simulink model "uavsim"  (R2024b)
settings: Solver=ode23  StartTime=0.0  StopTime=60  RelTol=1e-3  EnableMultiTasking=on
values from neighbouring files (symbols this model uses):
  P = real(.5*P + .5*P')    [ekf_driver.m]    (also in init_uavsim_params.m = []; load_uavsim.m = compute_autopilot_gains(models,P))
undefined symbols (not defined in the file or in its folder): uavsim_control, uavsim_display, uavsim_estimates, uavsim_forces_moments, uavsim_kin_dyn, uavsim_logging, uavsim_sensors, uavsim_trajectory_control, uavsim_truth_feedback, uavsim_wind
libraries: simulink x6
settings Model: Creator=bartojd1  LastModifiedBy=yeboaka1
settings SolverCC: AlgebraicLoopSolver=TrustRegion
settings DataIOCC: LimitDataPoints=on  SaveFormat=Array  SignalLoggingSaveFormat=ModelDataLogs  SaveOutput=off  SignalLogging=off  SaveTime=off  ReturnWorkspaceOutputs=off
settings OptimizationCC: ExpressionDepthLimit=2147483647  LifeSpan=inf
settings DebuggingCC: SolverPrmCheckMsg=warning  FcnCallInpInsideContextMsg=warning  UnconnectedInputMsg=warning  UnconnectedOutputMsg=warning  UnconnectedLineMsg=warning  StateNameClashWarn=warning  SFUnexpectedBacktrackingDiag=warning  SFNoUnconditionalDefaultTransitionDiag=warning  SFExecutionAtInitializationDiag=none  ArithmeticOperatorsInVariantConditions=warning
settings HardwareCC: ProdBitPerPointer=32  ProdBitPerSizeT=32  ProdBitPerPtrDiffT=32  ProdLargestAtomicFloat=None  ProdIntDivRoundTo=Undefined  ProdEndianess=Unspecified  ProdWordSize=32  ProdHWDeviceType=32-bit Generic
settings ModelReferenceCC: PropagateSignalLabelsOutOfModel=off
settings SFSimCC: SimUseLocalCustomCode=off  CustomCodeUndefinedFunction=UseInterfaceOnly
settings RTWCC: RTWUseLocalCustomCode=off  GPUComputeCapability=3.5
settings CodeAppCC: StateflowObjectComments=on
settings GRTTargetCC: TargetLangStandard=C89/C90 (ANSI)  CombineOutputUpdateFcns=off  GRTInterface=on
settings ConfigComp: CovMetricSettings=dw  CovSaveCumulativeToWorkspaceVar=on  CovSaveSingleToWorkspaceVar=on  CovExternalEMLEnable=off  CovSFcnEnable=off

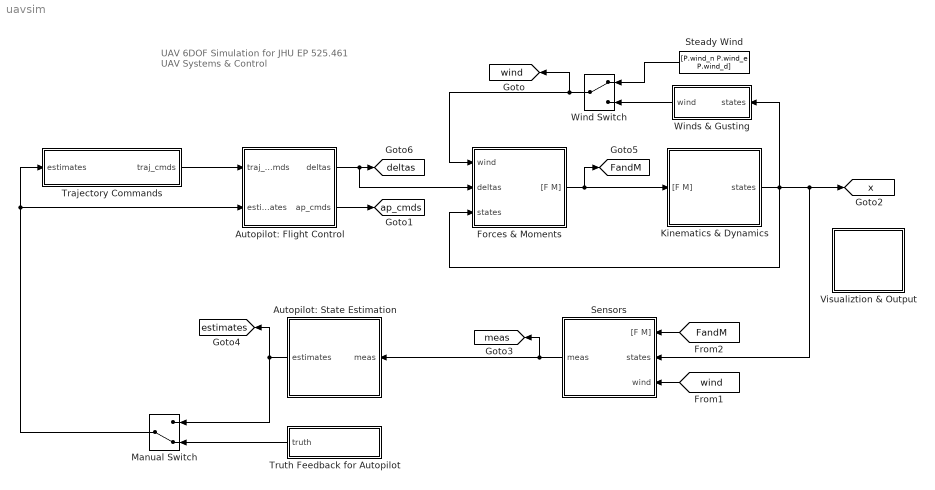
== system uavsim ==
  note: UAV 6DOF Simulation
      | for JHU EP 525.461
      | UAV Systems & Control
  Autopilot: Flight Control : Subsystem
  Autopilot: State Estimation : Subsystem
  Forces & Moments : Subsystem
  Kinematics & Dynamics : Subsystem
  Manual Switch : ManualSwitch  CurrentSetting=0
  Sensors : Subsystem
  Steady Wind : Constant  Value=[P.wind_n P.wind_e P.wind_d]
  Trajectory Commands : Subsystem
  Truth Feedback for Autopilot : Subsystem
  Visualiztion & Output : Subsystem
  Wind Switch : ManualSwitch
  Winds & Gusting : Subsystem
  tag scope: FandM=global, ap_cmds=global, deltas=global, estimates=global, meas=global, wind=global, x=global
  wires:
  Kinematics & Dynamics/1(states) -> Forces & Moments/3(states), Winds & Gusting/1(states), [x], Sensors/2(states)
  Forces & Moments/1("[F M]") -> Kinematics & Dynamics/1("[F M]"), [FandM]
  Sensors/1(meas) -> Autopilot: State Estimation/1(meas), [meas]
  [wind] -> Sensors/3(wind)
  Autopilot: Flight Control/2(ap_cmds) -> [ap_cmds]
  [FandM] -> Sensors/1("[F M]")
  Trajectory Commands/1(" traj_cmds") -> Autopilot: Flight Control/1(traj_cmds)
  Winds & Gusting/1(wind) -> Wind Switch/2
  Wind Switch/1 -> Forces & Moments/1("wind  "), [wind]
  Steady Wind/1 -> Wind Switch/1
  Autopilot: Flight Control/1(deltas) -> [deltas], Forces & Moments/2(deltas)
  Autopilot: State Estimation/1(estimates) -> Manual Switch/1, [estimates]
  Truth Feedback for Autopilot/1(truth) -> Manual Switch/2
  Manual Switch/1 -> Autopilot: Flight Control/2(estimates), Trajectory Commands/1(estimates)

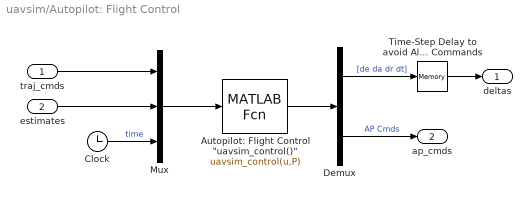
== system uavsim/Autopilot: Flight Control ==
  traj_cmds : Inport
  estimates : Inport  Port=2
  "Autopilot: Flight Control \"uavsim_control()\"" : MATLABFcn  MATLABFcn=uavsim_control(u,P)  OutputDimensions=4+9  SampleTime="P.Ts     % Autopilot at 100Hz"
  Clock : Clock
  Demux : Demux  Outputs=[4;9]
  Mux : Mux  Inputs=3
  Time-Step Delay to avoid Algepraic Loop I.C.: Trim Commands : Memory  InitialCondition=[P.delta_e0 P.delta_a0 P.delta_r0 P.delta_t0]'
  deltas : Outport
  ap_cmds : Outport  Port=2
  wires:
  Clock/1 -> Mux/3  "time"
  "Autopilot: Flight Control \"uavsim_control()\""/1 -> Demux/1
  Mux/1 -> "Autopilot: Flight Control \"uavsim_control()\""/1
  estimates/1 -> Mux/2
  traj_cmds/1 -> Mux/1
  Demux/2 -> ap_cmds/1  "AP Cmds"
  Demux/1 -> Time-Step Delay to avoid Algepraic Loop I.C.: Trim Commands/1  "[de da dr dt]"
  Time-Step Delay to avoid Algepraic Loop I.C.: Trim Commands/1 -> deltas/1

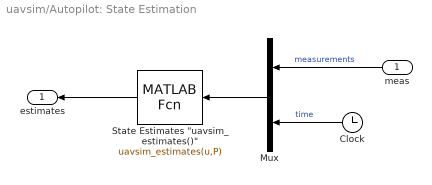
== system uavsim/Autopilot: State Estimation ==
  meas : Inport
  Clock : Clock
  Mux : Mux  Inputs=2
  "State Estimates \"uavsim_estimates()\"" : MATLABFcn  MATLABFcn=uavsim_estimates(u,P)  OutputDimensions=23  SampleTime="P.Ts   % Autopilot at 100 Hz"
  estimates : Outport
  wires:
  meas/1 -> Mux/1  "measurements"
  Mux/1 -> "State Estimates \"uavsim_estimates()\""/1
  Clock/1 -> Mux/2  "time"
  "State Estimates \"uavsim_estimates()\""/1 -> estimates/1

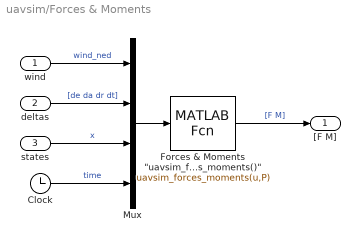
== system uavsim/Forces & Moments ==
  "wind  " : Inport
  deltas : Inport  Port=2
  states : Inport  Port=3
  Clock : Clock
  "Forces & Moments \"uavsim_forces_moments()\"" : MATLABFcn  MATLABFcn=uavsim_forces_moments(u,P)  OutputDimensions=3+3 % (3 forces), (3 moments)
  Mux : Mux
  "[F M]" : Outport
  wires:
  "Forces & Moments \"uavsim_forces_moments()\""/1 -> "[F M]"/1  "[F M]"
  Mux/1 -> "Forces & Moments \"uavsim_forces_moments()\""/1
  Clock/1 -> Mux/4  "time"
  "wind  "/1 -> Mux/1  "wind_ned"
  deltas/1 -> Mux/2  "[de da dr dt]"
  states/1 -> Mux/3  "x"

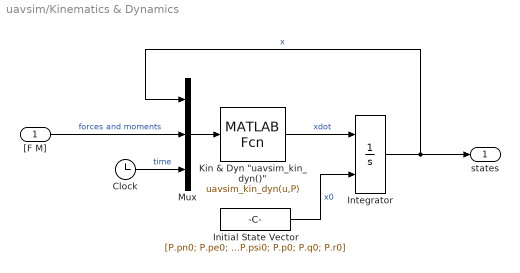
== system uavsim/Kinematics & Dynamics ==
  "[F M]" : Inport
  Clock : Clock
  Initial State Vector : Constant  Value=[P.pn0; P.pe0; P.pd0; P.u0; P.v0; P.w0; P.phi0; P.theta0; P.psi0; P.p0; P.q0; P.r0]
  Integrator : Integrator  InitialConditionSource=external
  "Kin & Dyn \"uavsim_kin_dyn()\"" : MATLABFcn  MATLABFcn=uavsim_kin_dyn(u,P)  OutputDimensions="12    % # of states"
  Mux : Mux  Inputs=3
  states : Outport
  wires:
  Integrator/1 -> Mux/1, states/1  "x"
  Mux/1 -> "Kin & Dyn \"uavsim_kin_dyn()\""/1
  "Kin & Dyn \"uavsim_kin_dyn()\""/1 -> Integrator/1  "xdot"
  "[F M]"/1 -> Mux/2  "forces and moments"
  Initial State Vector/1 -> Integrator/2  "x0"
  Clock/1 -> Mux/3  "time"

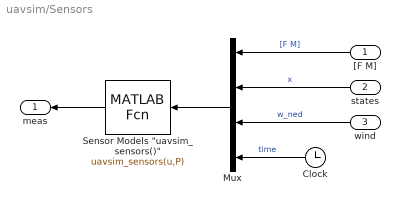
== system uavsim/Sensors ==
  "[F M]" : Inport
  states : Inport  Port=2
  wind : Inport  Port=3
  Clock : Clock
  Mux : Mux
  "Sensor Models \"uavsim_sensors()\"" : MATLABFcn  MATLABFcn=uavsim_sensors(u,P)  OutputDimensions=18  SampleTime=P.Ts
  meas : Outport
  wires:
  Mux/1 -> "Sensor Models \"uavsim_sensors()\""/1
  "Sensor Models \"uavsim_sensors()\""/1 -> meas/1
  Clock/1 -> Mux/4  "time"
  "[F M]"/1 -> Mux/1  "[F M]"
  states/1 -> Mux/2  "x"
  wind/1 -> Mux/3  "w_ned"

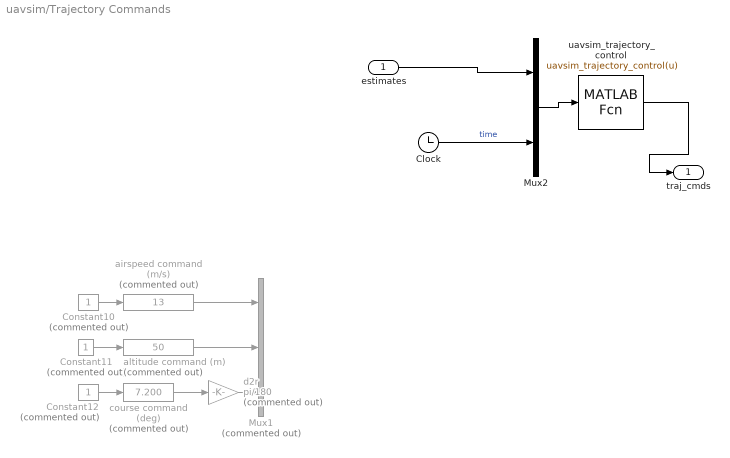
== system uavsim/Trajectory Commands ==
  estimates : Inport
  Clock : Clock
  Constant10 : Constant  Commented=on
  Constant11 : Constant  Commented=on
  Constant12 : Constant  Commented=on
  Mux1 : Mux  Commented=on  Inputs=3
  Mux2 : Mux  Inputs=2
  airspeed command (m/s) : simulink/Math Operations/Slider Gain  Commented=on  gain=13  low=5  high=18
  altitude command (m) : simulink/Math Operations/Slider Gain  Commented=on  gain=50  low=0  high=100
  course command (deg) : simulink/Math Operations/Slider Gain  Commented=on  gain=7.200  low=-360  high=360
  d2r : Gain  Commented=on  Gain=pi/180
  uavsim_trajectory_control : MATLABFcn  MATLABFcn=uavsim_trajectory_control(u)  OutputDimensions=3  SampleTime="P.Ts     % Autopilot at 100Hz"
  " traj_cmds" : Outport
  wires:
  Constant10/1 -> airspeed command (m/s)/1
  Constant11/1 -> altitude command (m)/1
  Constant12/1 -> course command (deg)/1
  course command (deg)/1 -> d2r/1
  altitude command (m)/1 -> Mux1/2
  airspeed command (m/s)/1 -> Mux1/1
  d2r/1 -> Mux1/3
  uavsim_trajectory_control/1 -> " traj_cmds"/1
  estimates/1 -> Mux2/1
  Clock/1 -> Mux2/2  "time"
  Mux2/1 -> uavsim_trajectory_control/1

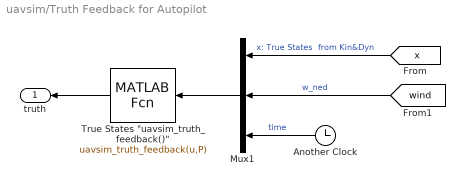
== system uavsim/Truth Feedback for Autopilot ==
  Another Clock : Clock
  Mux1 : Mux  Inputs=3
  "True States \"uavsim_truth_feedback()\"" : MATLABFcn  MATLABFcn=uavsim_truth_feedback(u,P)  OutputDimensions=23  SampleTime="P.Ts   % Autopilot at 100 Hz"
  truth : Outport
  wires:
  Mux1/1 -> "True States \"uavsim_truth_feedback()\""/1
  [x] -> Mux1/1  "x: True States  from Kin&Dyn"
  [wind] -> Mux1/2  "w_ned"
  Another Clock/1 -> Mux1/3  "time"
  "True States \"uavsim_truth_feedback()\""/1 -> truth/1

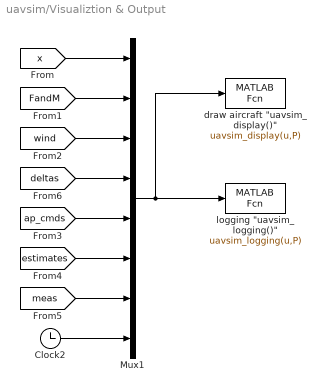
== system uavsim/Visualiztion & Output ==
  Clock2 : Clock
  Mux1 : Mux  Inputs=8
  "draw aircraft \"uavsim_display()\"" : MATLABFcn  MATLABFcn=uavsim_display(u,P)  OutputDimensions=0  SampleTime=P.Tvis
  "logging \"uavsim_logging()\"" : MATLABFcn  MATLABFcn=uavsim_logging(u,P)  OutputDimensions=0  SampleTime=P.Tlog
  wires:
  [FandM] -> Mux1/2
  [wind] -> Mux1/3
  Mux1/1 -> "logging \"uavsim_logging()\""/1, "draw aircraft \"uavsim_display()\""/1
  [x] -> Mux1/1
  [deltas] -> Mux1/4
  [ap_cmds] -> Mux1/5
  [estimates] -> Mux1/6
  [meas] -> Mux1/7
  Clock2/1 -> Mux1/8

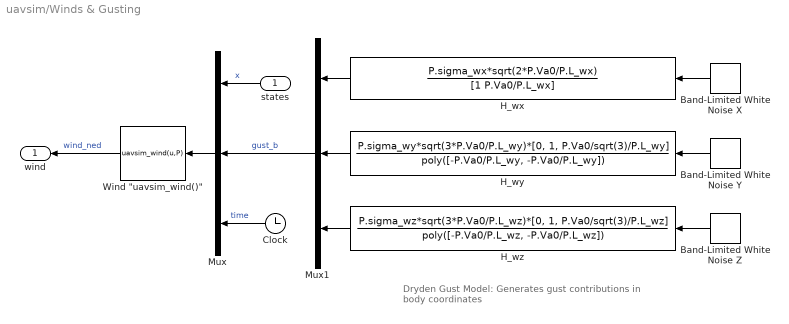
== system uavsim/Winds & Gusting ==
  note: Dryden Gust Model:
      | Generates gust contributions in body coordinates
  states : Inport
  Band-Limited White Noise X : simulink/Sources/Band-Limited White Noise  Cov=[1]  Ts=P.Ts  seed=round(1e9*rand)
  Band-Limited White Noise Y : simulink/Sources/Band-Limited White Noise  Cov=[1]  Ts=P.Ts  seed=round(1e9*rand)
  Band-Limited White Noise Z : simulink/Sources/Band-Limited White Noise  Cov=[1]  Ts=P.Ts  seed=round(1e9*rand)
  Clock : Clock
  H_wx : TransferFcn  Numerator=P.sigma_wx*sqrt(2*P.Va0/P.L_wx)  Denominator=[1 P.Va0/P.L_wx]
  H_wy : TransferFcn  Numerator=P.sigma_wy*sqrt(3*P.Va0/P.L_wy)*[0, 1, P.Va0/sqrt(3)/P.L_wy]  Denominator=poly([-P.Va0/P.L_wy, -P.Va0/P.L_wy])
  H_wz : TransferFcn  Numerator=P.sigma_wz*sqrt(3*P.Va0/P.L_wz)*[0, 1, P.Va0/sqrt(3)/P.L_wz]  Denominator=poly([-P.Va0/P.L_wz, -P.Va0/P.L_wz])
  Mux : Mux  Inputs=3
  Mux1 : Mux  Inputs=3
  "Wind \"uavsim_wind()\"" : MATLABFcn  MATLABFcn=uavsim_wind(u,P)  OutputDimensions=3
  wind : Outport
  wires:
  Mux/1 -> "Wind \"uavsim_wind()\""/1
  "Wind \"uavsim_wind()\""/1 -> wind/1  "wind_ned"
  states/1 -> Mux/1  "x"
  Clock/1 -> Mux/3  "time"
  Mux1/1 -> Mux/2  "gust_b"
  H_wx/1 -> Mux1/1
  H_wy/1 -> Mux1/2
  H_wz/1 -> Mux1/3
  Band-Limited White Noise X/1 -> H_wx/1
  Band-Limited White Noise Y/1 -> H_wy/1
  Band-Limited White Noise Z/1 -> H_wz/1
